simulink model "model2"  (Simulink 7.5)
settings: Solver=ode45  StartTime=0.0  StopTime=inf  RelTol=1e-3
settings Model: Creator=paris  LastModifiedBy=paris

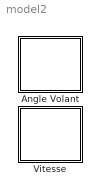
== system model2 ==
  Angle Volant : Stateflow chart  TreatAsAtomicUnit=on
  Vitesse : Stateflow chart  TreatAsAtomicUnit=on

== stateflow chart Angle Volant ==
  state volant [parallel]
    settings: executionOrder=1
    state droite
      %entry: ml.addState('Volant.droite',ml.timecode,ml.qs,'qs')
      state droiteRapide
        %entry: ml.sendState('V.DR',ml.timecode,ml.exportBot,'toto@w7-paris','stateflow@w7-paris/toto')%
      state droiteLente
      (default) -> droiteRapide
      droiteRapide -> droiteLente : [ml.vitesse > 40]
      droiteLente -> droiteRapide : [ml.vitesse < 40]
    state toutdroit
      %entry: ml.addState('Volant.todoRecto',ml.timecode,ml.qs,'qs')
    state gauche
      %entry: ml.addState('Volant.gauche',ml.timecode,ml.qs,'qs')
    (default) -> toutdroit
    toutdroit -> droite [order 1] : [ml.volant > 10]
    droite -> toutdroit : [ml.volant < 10]
    gauche -> toutdroit : [ml.volant > -10]
    toutdroit -> gauche [order 2] : [ml.volant < -10]
  state vitesse [parallel]
    settings: executionOrder=2
    state tropVite
      %entry: ml.addState('Vitesse.tropVite',ml.timecode,ml.qs2,'qs2')
    state normal
      %entry: ml.addState('Vitesse.normalVite',ml.timecode,ml.qs2,'qs2')
    (default) -> normal
    normal -> tropVite : [ml.vitesse > 50]
    tropVite -> normal : [ml.vitesse < 50]

== stateflow chart Vitesse ==
  state lent
  state rapide
  (default) -> lent
  lent -> rapide : [ml.vitesse>=30]
  rapide -> lent : [ml.vitesse<30]
